simulink model "CoVM"  (R2018a)
settings: configuration reference "cs_ert" (kept outside this file)
settings Model: DataDictionary=CoVM.sldd  Creator=zhoutinglin  LastModifiedBy=zhoutinglin

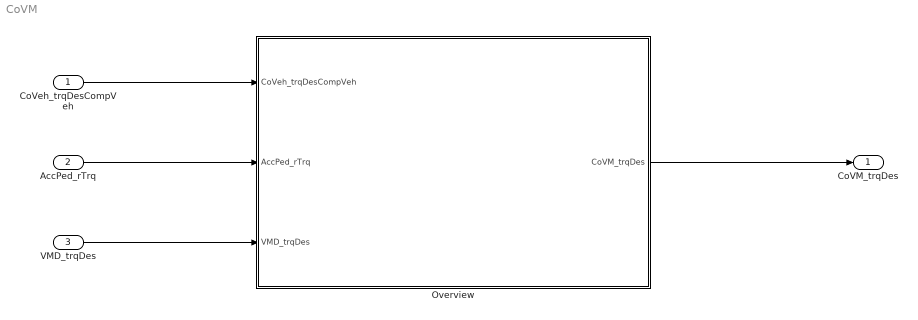
== system CoVM ==
  CoVeh_trqDesCompVeh : Inport
  AccPed_rTrq : Inport  Port=2
  VMD_trqDes : Inport  Port=3
  Overview : Subsystem
  CoVM_trqDes : Outport
  wires:
  CoVeh_trqDesCompVeh/1 -> Overview/1(CoVeh_trqDesCompVeh)
  AccPed_rTrq/1 -> Overview/2(AccPed_rTrq)
  VMD_trqDes/1 -> Overview/3(VMD_trqDes)
  Overview/1(CoVM_trqDes) -> CoVM_trqDes/1

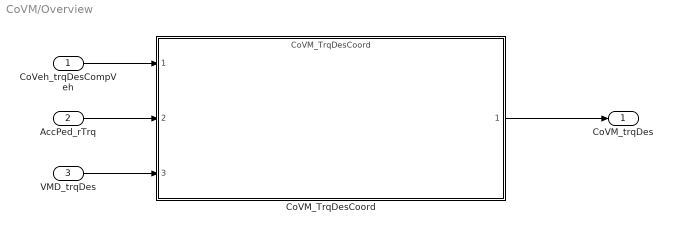
== system CoVM/Overview ==
  CoVeh_trqDesCompVeh : Inport
  AccPed_rTrq : Inport  Port=2
  VMD_trqDes : Inport  Port=3
  CoVM_TrqDesCoord : ModelReference  ModelNameDialog=CoVM_TrqDesCoord  SimulationMode=Normal  ModelReferenceVersion=1.49
  CoVM_trqDes : Outport
  wires:
  CoVeh_trqDesCompVeh/1 -> CoVM_TrqDesCoord/1
  AccPed_rTrq/1 -> CoVM_TrqDesCoord/2
  VMD_trqDes/1 -> CoVM_TrqDesCoord/3
  CoVM_TrqDesCoord/1 -> CoVM_trqDes/1
